simulink model "Power_Forcasting_SOC"  (R2024a)
settings: Solver=VariableStepAuto  StartTime=0.0  StopTime=2154  RelTol=1e-3
undefined symbols (not defined in the file or in its folder): DiscIntNeverNeededParam
libraries: slpidlib x2, dspstat3 x2, simulink x2
settings Model: Creator=ezeki  LastModifiedBy=ezeki

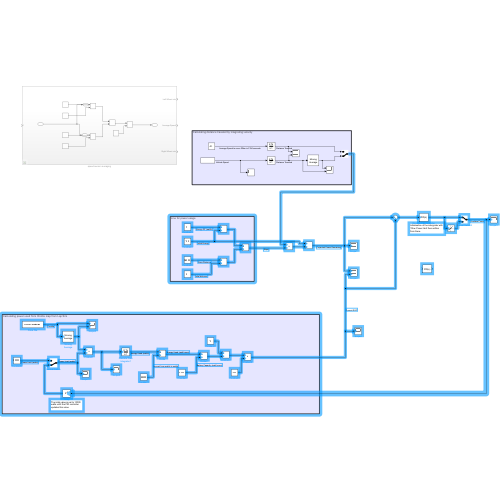
[thumbnail: Simulink's stored preview of the top-level diagram]
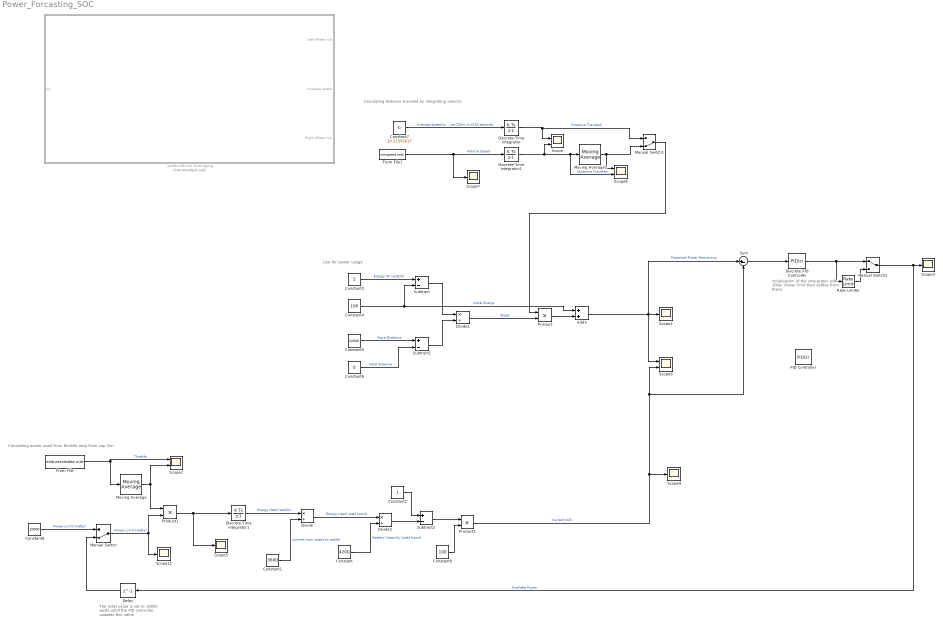
== system Power_Forcasting_SOC ==
  note: Calculating distance traveled by integrating velocity
  note: Calculating power used from throttle map from Lap Sim
  note: Line for power usage
  note: Initialisation of the intergrater with 10kw. Power limit then settles from there.
  note: The inital value is set to 10000 watts untill the PID controller updates this value
  Add3 : Sum
  Constant : Constant  Value=4200
  Constant1 : Constant  Value=3600
  Constant2 : Constant
  Constant3 : Constant  Value=5
  Constant4 : Constant  Value=100
  Constant5 : Constant  Value=22000
  Constant6 : Constant  Value=0
  Constant7 : Constant  Value=10.21355617
  Constant8 : Constant  Value=10000
  Constant9 : Constant  Value=100
  Delay : Delay  DelayLength=1  InitialCondition=10000
  Discrete PID Controller : slpidlib/PID Controller  Controller=PID  Form=Parallel  TimeDomain=Discrete-time  UseExternalTs=off  SampleTime=-1  IntegratorMethod=Forward Euler  FilterMethod=Forward Euler  ControllerParametersSource=internal  P=-420  I=0.042  UseKiTs=off  D=21000  UseExternalDerivativeSource=off  N=0.01  UseFilter=on  TunerSelectOption=Transfer Function Based (PID Tuner App)  InitialConditionSource=internal  InitialConditionForIntegrator=10000  InitialConditionForFilter=0  DifferentiatorICPrevScaledInput=0  ExternalReset=none  TrackingMode=off  Kt=1  LimitOutput=off  SatLimitsSource=internal  UpperSaturationLimit=inf  LowerSaturationLimit=-inf  LinearizeAsGain=off  AntiWindupMode=none  Kb=1  LimitIntegrator=off  UpperIntegratorSaturationLimit=inf  LowerIntegratorSaturationLimit=-inf  POutMin=[]  POutMax=[]  IOutMin=[]  IOutMax=[]  DOutMin=[]  DOutMax=[]  NOutMin=[]  NOutMax=[]  SumOutMin=[]  SumOutMax=[]  SaturationOutMin=[]  SaturationOutMax=[]  PParamMin=[]  PParamMax=[]  IParamMin=[]  IParamMax=[]  DParamMin=[]  DParamMax=[]  NParamMin=[]  NParamMax=[]  KbParamMin=[]  KbParamMax=[]  KtParamMin=[]  KtParamMax=[]  KbOutMin=[]  KbOutMax=[]  KtOutMin=[]  KtOutMax=[]  IntegratorOutMin=[]  IntegratorOutMax=[]  FilterOutMin=[]  FilterOutMax=[]  SumI1OutMin=[]  SumI1OutMax=[]  SumI2OutMin=[]  SumI2OutMax=[]  SumI3OutMin=[]  SumI3OutMax=[]  SumI4OutMin=[]  SumI4OutMax=[]  SumDOutMin=[]  SumDOutMax=[]  DifferentiatorOutMin=[]  DifferentiatorOutMax=[]  FilterDiffOutCoefMin=[]  FilterDiffOutCoefMax=[]  ReciprocalOutMin=[]  ReciprocalOutMax=[]  SumDenOutMin=[]  SumDenOutMax=[]  SumNumOutMin=[]  SumNumOutMax=[]  DivideOutMin=[]  DivideOutMax=[]  UdiffTsProdOutMin=[]  UdiffTsProdOutMax=[]  NTsProdOutMin=[]  NTsProdOutMax=[]  UintegralTsProdOutMin=[]  UintegralTsProdOutMax=[]  UngainTsProdOutMin=[]  UngainTsProdOutMax=[]  ClampingZeroOutDataTypeStr=Inherit: Inherit via back propagation  ClampingZeroOutMin=[]  ClampingZeroOutMax=[]  FilterDenConstantOutDataTypeStr=Inherit: Inherit via back propagation  FilterDenConstantOutMin=[]  FilterDenConstantOutMax=[]  PCopyOutDataTypeStr=Inherit: Inherit via back propagation  PCopyOutMin=[]  PCopyOutMax=[]  NCopyOutDataTypeStr=Inherit: Inherit via back propagation  NCopyOutMin=[]  NCopyOutMax=[]  IntegratorContinuousStateAttributes=''  IntegratorStateMustResolveToSignalObject=off  IntegratorRTWStateStorageClass=Auto  FilterContinuousStateAttributes=''  FilterStateMustResolveToSignalObject=off  FilterRTWStateStorageClass=Auto  ParallelPVariant=InternalParameters  IdealPVariant=Disabled  IVariant=InternalParameters  DVariant=InternalParameters  IntegratorVariant=Discrete  SatVariant=Disabled  AWVariant=Passthrough  PCopyVariant=Disabled  TRVariant=Disabled  FdbkBlocksVariant=Forward  IdealPFdbkVariant=Disabled  SatFdbkVariant=Disabled  DerivativeFilterVariant=ForwardEulerFilter  NVariant=InternalParameters  NCopyVariant=Disabled  FilterICVariant=InternalICsFilter  IntegratorICVariant=InternalICs  ExternalResetVariant=Disabled  TRSumVariant=Passthrough  SumFdbkVariant=Disabled  SumVariant=Sum_PID  TsampFilterVariant=InternalTs  TsampNgainVariant=Passthrough  TsampIntegralVariant=Disabled_SignalSpec  ExternalSaturationOutDataTypeStr=Inherit: Same as second input  DerivativeSourceVariant=ErrorSignal
      settings: LibrarySourceBlock=simulink/Discrete/Discrete PID Controller
  Discrete-Time Integrator : DiscreteIntegrator  SampleTime=0.01  ICPrevOutput=DiscIntNeverNeededParam  ICPrevScaledInput=DiscIntNeverNeededParam
  Discrete-Time Integrator1 : DiscreteIntegrator  SampleTime=0.01  ICPrevOutput=DiscIntNeverNeededParam  ICPrevScaledInput=DiscIntNeverNeededParam
  Discrete-Time Integrator2 : DiscreteIntegrator  SampleTime=0.01  ICPrevOutput=DiscIntNeverNeededParam  ICPrevScaledInput=DiscIntNeverNeededParam
  Divide : Product  Inputs=*/
  Divide1 : Product  Inputs=*/
  Divide2 : Product  Inputs=*/
  From File : FromFile  FileName=endurancedata.mat  SampleTime=0.01
  From File1 : FromFile  FileName=simspeed.mat  SampleTime=0.01
  Manual Switch : ManualSwitch  CurrentSetting=0
  Manual Switch1 : ManualSwitch  CurrentSetting=0
  Manual Switch2 : ManualSwitch
  Moving Average : dspstat3/Moving Average  Method=Sliding window  ForgettingFactorPort=off  SpecifyWindowLength=on  WindowLength=1000  OverlapLength=999  AllowArbitraryInputLength=off  ForgettingFactor=0.9  SimulateUsing=Interpreted execution
  Moving Average1 : dspstat3/Moving Average  Method=Sliding window  ForgettingFactorPort=off  SpecifyWindowLength=on  WindowLength=1000  OverlapLength=999  AllowArbitraryInputLength=off  ForgettingFactor=0.9  SimulateUsing=Interpreted execution
  PID Controller : slpidlib/PID Controller  Controller=PID  Form=Parallel  TimeDomain=Continuous-time  UseExternalTs=off  SampleTime=-1  IntegratorMethod=Forward Euler  FilterMethod=Forward Euler  ControllerParametersSource=internal  P=-10.  I=0.001  UseKiTs=off  D=500  UseExternalDerivativeSource=off  N=0.01  UseFilter=on  TunerSelectOption=Transfer Function Based (PID Tuner App)  InitialConditionSource=internal  InitialConditionForIntegrator=10000  InitialConditionForFilter=0  DifferentiatorICPrevScaledInput=0  ExternalReset=none  TrackingMode=off  Kt=1  LimitOutput=off  SatLimitsSource=internal  UpperSaturationLimit=inf  LowerSaturationLimit=-inf  LinearizeAsGain=on  AntiWindupMode=none  Kb=1  LimitIntegrator=off  UpperIntegratorSaturationLimit=inf  LowerIntegratorSaturationLimit=-inf  POutMin=[]  POutMax=[]  IOutMin=[]  IOutMax=[]  DOutMin=[]  DOutMax=[]  NOutMin=[]  NOutMax=[]  SumOutMin=[]  SumOutMax=[]  SaturationOutMin=[]  SaturationOutMax=[]  PParamMin=[]  PParamMax=[]  IParamMin=[]  IParamMax=[]  DParamMin=[]  DParamMax=[]  NParamMin=[]  NParamMax=[]  KbParamMin=[]  KbParamMax=[]  KtParamMin=[]  KtParamMax=[]  KbOutMin=[]  KbOutMax=[]  KtOutMin=[]  KtOutMax=[]  IntegratorOutMin=[]  IntegratorOutMax=[]  FilterOutMin=[]  FilterOutMax=[]  SumI1OutMin=[]  SumI1OutMax=[]  SumI2OutMin=[]  SumI2OutMax=[]  SumI3OutMin=[]  SumI3OutMax=[]  SumI4OutMin=[]  SumI4OutMax=[]  SumDOutMin=[]  SumDOutMax=[]  DifferentiatorOutMin=[]  DifferentiatorOutMax=[]  FilterDiffOutCoefMin=[]  FilterDiffOutCoefMax=[]  ReciprocalOutMin=[]  ReciprocalOutMax=[]  SumDenOutMin=[]  SumDenOutMax=[]  SumNumOutMin=[]  SumNumOutMax=[]  DivideOutMin=[]  DivideOutMax=[]  UdiffTsProdOutMin=[]  UdiffTsProdOutMax=[]  NTsProdOutMin=[]  NTsProdOutMax=[]  UintegralTsProdOutMin=[]  UintegralTsProdOutMax=[]  UngainTsProdOutMin=[]  UngainTsProdOutMax=[]  ClampingZeroOutDataTypeStr=Inherit: Inherit via back propagation  ClampingZeroOutMin=[]  ClampingZeroOutMax=[]  FilterDenConstantOutDataTypeStr=Inherit: Inherit via back propagation  FilterDenConstantOutMin=[]  FilterDenConstantOutMax=[]  PCopyOutDataTypeStr=Inherit: Inherit via back propagation  PCopyOutMin=[]  PCopyOutMax=[]  NCopyOutDataTypeStr=Inherit: Inherit via back propagation  NCopyOutMin=[]  NCopyOutMax=[]  IntegratorContinuousStateAttributes=''  IntegratorStateMustResolveToSignalObject=off  IntegratorRTWStateStorageClass=Auto  FilterContinuousStateAttributes=''  FilterStateMustResolveToSignalObject=off  FilterRTWStateStorageClass=Auto  ParallelPVariant=InternalParameters  IdealPVariant=Disabled  IVariant=InternalParameters  DVariant=InternalParameters  IntegratorVariant=Continuous  SatVariant=Disabled  AWVariant=Passthrough  PCopyVariant=Disabled  TRVariant=Disabled  FdbkBlocksVariant=Forward  IdealPFdbkVariant=Disabled  SatFdbkVariant=Disabled  DerivativeFilterVariant=ContFilter  NVariant=InternalParameters  NCopyVariant=Disabled  FilterICVariant=InternalICsFilter  IntegratorICVariant=InternalICs  ExternalResetVariant=Disabled  TRSumVariant=Passthrough  SumFdbkVariant=Disabled  SumVariant=Sum_PID  TsampFilterVariant=InternalTs  TsampNgainVariant=Passthrough  TsampIntegralVariant=Disabled_SignalSpec  ExternalSaturationOutDataTypeStr=Inherit: Same as second input  DerivativeSourceVariant=ErrorSignal
  Product : Product
  Product1 : Product
  Product2 : Product
  Rate Limiter : RateLimiter  RisingSlewLimit=10  FallingSlewLimit=-10  SampleTimeMode=inherited
  Scope{,2,6,8} (4 alike) : Scope  NumInputPorts=2
  Scope{1,3..5,7,11} (6 alike) : Scope
  Subtract : Sum  Inputs=+-
  Subtract1 : Sum  Inputs=+-
  Subtract2 : Sum  Inputs=+-
  Sum : Sum  Inputs=|+-
  speed sensor averaging : Subsystem  Commented=on
  wires:
  Discrete-Time Integrator/1 -> Manual Switch1/1, Scope/1  "Distance Traveled"
  Constant3/1 -> Subtract/1  "Energy SF (watt/h)"
  Constant4/1 -> Add3/1, Subtract/2  "Initial Energy"
  Constant6/1 -> Subtract1/2  "Intial distance"
  Constant5/1 -> Subtract1/1  "Race Distance"
  Subtract/1 -> Divide1/1
  Subtract1/1 -> Divide1/2
  Divide1/1 -> Product/2  "Slope"
  Product/1 -> Add3/2
  Add3/1 -> Scope6/1, Sum/1, Scope1/1  "Projected Power Remaining"
  From File/1 -> Scope2/1, Moving Average/1  "Throttle"
  Manual Switch/1 -> Scope11/1, Product1/2  "Power Limit (watts)"
  Product1/1 -> Scope5/1, Discrete-Time Integrator1/1
  Divide/1 -> Divide2/1  "Energy Used (watt hours)"
  Constant7/1 -> Discrete-Time Integrator/1  "Average Speed to cover 22km in 2154 seconds"
  Constant/1 -> Divide2/2  "Battery Capacity (watt hours)"
  Product2/1 -> Scope4/1, Sum/2, Scope6/2  "Current SOC"
  Discrete-Time Integrator1/1 -> Divide/1  "Energy Used (watt/s)"
  Constant1/1 -> Divide/2  "convert from watt/s to watt/h"
  Constant8/1 -> Manual Switch/1  "Power Limit (watts)"
  Sum/1 -> Discrete PID Controller/1
  Delay/1 -> Manual Switch/2
  Discrete PID Controller/1 -> Manual Switch2/1, Rate Limiter/1
  Moving Average/1 -> Scope2/2, Product1/1
  From File1/1 -> Scope7/1, Discrete-Time Integrator2/1  "Vehicle Speed"
  Discrete-Time Integrator2/1 -> Scope/2, Scope8/2, Moving Average1/1  "Distance Traveled"
  Manual Switch2/1 -> Delay/1, Scope3/1  "Availabe Power"
  Rate Limiter/1 -> Manual Switch2/2
  Manual Switch1/1 -> Product/1
  Moving Average1/1 -> Scope8/1, Manual Switch1/2
  Divide2/1 -> Subtract2/2
  Constant2/1 -> Subtract2/1
  Subtract2/1 -> Product2/1
  Constant9/1 -> Product2/2

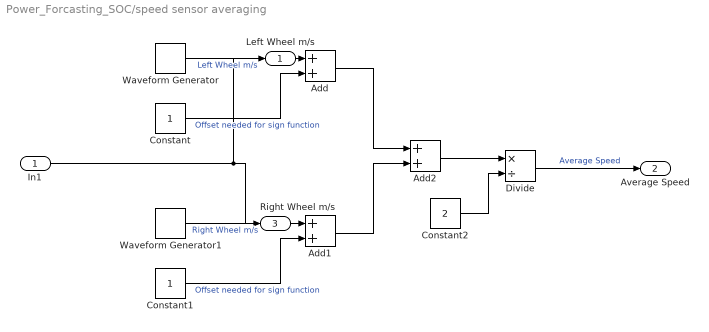
== system Power_Forcasting_SOC/speed sensor averaging ==
  In1 : Inport
  Add : Sum
  Add1 : Sum
  Add2 : Sum
  Constant : Constant
  Constant1 : Constant
  Constant2 : Constant  Value=2
  Divide : Product  Inputs=*/
  Waveform Generator : simulink/Sources/Waveform Generator  OutMin=[]  OutMax=[]  OutDataTypeStr=double  SelectedSignal=1  Signals=sin('Amplitude',1,'Frequency',1,'Phase',0)  BlockNames=MultiportSwitch_9f863abd22c444e  SampleTime=0.1
  Waveform Generator1 : simulink/Sources/Waveform Generator  OutMin=[]  OutMax=[]  OutDataTypeStr=double  SelectedSignal=1  Signals=sin('Amplitude',1,'Frequency',1,'Phase',0)  BlockNames=MultiportSwitch_9f863abd22c444e  SampleTime=0.1
  Left Wheel m/s : Outport
  Average Speed : Outport  Port=2
  Right Wheel m/s : Outport  Port=3
  wires:
  In1/1 -> Add/1, Add1/1
  Add1/1 -> Add2/2
  Constant1/1 -> Add1/2  "Offset needed for sign function"
  Waveform Generator1/1 -> Right Wheel m/s/1  "Right Wheel m/s"
  Add/1 -> Add2/1
  Constant2/1 -> Divide/2
  Constant/1 -> Add/2  "Offset needed for sign function"
  Add2/1 -> Divide/1
  Waveform Generator/1 -> Left Wheel m/s/1  "Left Wheel m/s"
  Divide/1 -> Average Speed/1  "Average Speed"
